simulink model "QiMotorController_ModelReference"  (R2021b)
settings: Solver=FixedStepDiscrete  StartTime=0.0  StopTime=5  RelTol=1e-3
PreLoadFcn:
  | RTWConfigurationCB('preloadfcn', bdroot);
PostLoadFcn:
  | load('configuration/data_struct.mat');
  | load('configuration/fluxMaps_propMotor.mat');
  | load('configuration/parameterInit_PROP.mat');
  | load('configuration/parameterInit_PUMP.mat');
  | load('configuration/parameterInit_PITCH.mat');
  | load('configuration/parameterInit_TILT.mat');
  | %load('configuration/base_workspace_signal_definition.mat');
  | %load('resolvedatastores_to_baseworkspace_for_faster_simulation.mat');
model workspace (MAT data in the model file):
  ADC_CALIBRATION_SAMPLES : Simulink.Parameter (value not decoded)
  DEFAULT_RESOLVER_CONTROL_WORD : Simulink.Parameter (value not decoded)
  PLL_FREQUENCY : Simulink.Parameter (value not decoded)
  SIMULATION_OPTIONS : Simulink.Parameter (value not decoded)
  TARGET_CODE_GEN : Simulink.Parameter (value not decoded)
  Ts = 2.5e-07
symbols that are objects in the model workspace (value not decoded): PLL_FREQUENCY, TARGET_CODE_GEN
undefined symbols (not defined in the file): DEADTIME_NS__PITCH, DEADTIME_NS__PROP, DEADTIME_NS__PUMP, DEADTIME_NS__TILT, fIa_, fIb_, fIc_, fIdc_, fMotorEncoderFloat_, fMotorSensorSpeed_, fUa_, fUb_, fUc_, fUdc_, inbtilt, mdl_pitch_uiAPUFlags, mdl_pitch_uiFlags, modelData, oMot_, oOut_, opInputResolverData_, oPitch, oState_, PLANT_SPEED_QUADRATIC_COEFF__PUMP, POLE_PAIRS_INIT__PITCH, POLE_PAIRS_INIT__PROP, POLE_PAIRS_INIT__PUMP, POLE_PAIRS_INIT__TILT, PWM_FREQ_KHZ__PITCH, PWM_FREQ_KHZ__PROP, PWM_FREQ_KHZ__PUMP, R_PHASE_INIT__PITCH, R_PHASE_INIT__PROP, R_PHASE_INIT__TILT, R_PHASE_INIT_PLANT__PUMP, uiControlReadback_, uiGateDriverStatus_
libraries: simulink x51, spsSeriesRLCBranchLib x25, spsMosfetLib x24, powerlib_extras x24, spsCurrentMeasurementLib x17, spsVoltageMeasurementLib x17, spsPermanentMagnetSynchronousMachineLib x3, spsDCVoltageSourceLib x2, motorModelLibrary x2, slpidlib x2, cstblocks x1, spspowerguiLib x1
(part 2 of 5)

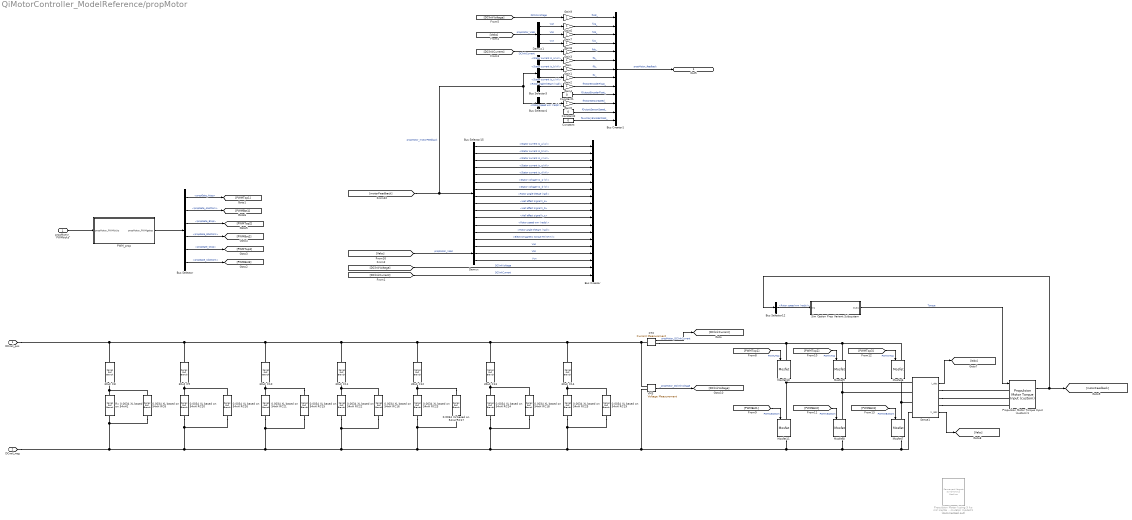
== system QiMotorController_ModelReference/propMotor ==
  propMotor_PWMticks : Inport
  0.0034 XL based on 54nH RC{8,15..19,26} (7 alike) : spsSeriesRLCBranchLib/Series RLC Branch  LConnTagsString=__new0  RConnTagsString=__new0  BranchType=R  Resistance=10000000  Inductance=33e-9  SetiL0=off  InitialCurrent=0  Capacitance=470e-6  Setx0=off  InitialVoltage=0  Measurements=None
  0.0034 XL based on 54nH RC{20..25} (6 alike) : spsSeriesRLCBranchLib/Series RLC Branch  LConnTagsString=__new0  RConnTagsString=__new0  BranchType=R  Resistance=0.0041  Inductance=33e-9  SetiL0=off  InitialCurrent=0  Capacitance=470e-6  Setx0=off  InitialVoltage=0  Measurements=None
  30uF C{8..10,12..14} (6 alike) : spsSeriesRLCBranchLib/Series RLC Branch  LConnTagsString=__new0  RConnTagsString=__new0  BranchType=C  Resistance=1  Inductance=1e-3  SetiL0=off  InitialCurrent=0  Capacitance=30e-6  Setx0=off  InitialVoltage=0  Measurements=Branch voltage and current
  30uF C11 : spsSeriesRLCBranchLib/Series RLC Branch  LConnTagsString=__new0  RConnTagsString=__new0  BranchType=C  Resistance=1  Inductance=1e-3  SetiL0=off  InitialCurrent=0  Capacitance=10e-6  Setx0=off  InitialVoltage=0  Measurements=Branch voltage and current
  Bus Creator : BusCreator  Inputs=19
  Bus Creator1 : BusCreator  Inputs=13  OutDataTypeStr=Bus: SAdcDataSingleIn_t
  Bus Selector : BusSelector  OutputSignals=propGate_Atop,propGate_Abottom,propGate_Btop,propGate_Bbottom,propGate_Ctop,propGate_Cbottom
  Bus Selector12 : BusSelector  OutputSignals=Rotor speed wm (rad/s)
  Bus Selector15 : BusSelector  OutputSignals=Stator current is_a (A),Stator current is_b (A),Stator current is_c (A),Stator current is_q (A),Stator current is_d (A),Stator voltage Vs_q (V),Stator voltage Vs_d (V),Rotor angle thetae (rad),Hall effect signal h_a,Hall effect signal h_b,Hall effect signal h_c,Rotor speed wm (rad/s),Rotor angle thetam (rad),Electromagnetic torque Te (N*m)
  Bus Selector3 : BusSelector  OutputSignals=Stator current is_a (A),Stator current is_b (A),Stator current is_c (A),Rotor angle thetam (rad)
  Bus Selector4 : BusSelector  OutputSignals=Rotor speed wm (rad/s)
  CT2 : spsCurrentMeasurementLib/Current Measurement  PhasorSimulation=off  OutputType=Complex  PSBequivalent=0
  Constant : Constant  Value=0  OutDataTypeStr=single
  Constant1 : Constant  Value=0  OutDataTypeStr=single
  Constant2 : Constant  Value=0  OutDataTypeStr=single
  Demux : Demux  Outputs=3
  Demux1 : Demux  Outputs=3
  Gain{,1..9} (10 alike) : Gain  OutDataTypeStr=single
  Mosfet{6..11} (6 alike) : spsMosfetLib/Mosfet  Ron=5e-3  Lon=0  Rd=0.01  Vfd=0  IC=0  Rs=1e5  Cs=inf  Measurements=on
  PWM_prop : Subsystem
  Propulsion Motor (using 5 kg m2 inertia consistent with the emulator model)1 : spsPermanentMagnetSynchronousMachineLib/Permanent Magnet Synchronous Machine  Commented=on  NbPhases=3  FluxDistribution=Sinusoidal  RotorType=Salient-pole  MechanicalLoad=Torque Tm  PresetModel=No  ShowDetailedParameters=on  MeasurementBus=off  Resistance=R_PHASE_INIT__PROP  Inductance=0  dqInductances=[160e-6 130e-6]  La=MOTOR_Ls  MachineConstant=Torque Constant (N.m / A_peak)  Flux=0.044127  VoltageCst=336.1575  TorqueCst=TORQUE_NM_PER_AMP_INIT__PROP  Flat=0  Mechanical=[0.89 0.005 POLE_PAIRS_INIT__PROP]  PolePairs=POLE_PAIRS_INIT__PROP  InitialConditions=[0,0,0,0]  InitialConditions5ph=[0 0 0 0 0 0]  RefAngle=Aligned with phase A axis (original Park)  IterativeDiscreteModel=Trapezoidal non iterative  TsBlock=Ts  TsPowergui=0
      link override From: GotoTag=tp8169b85b_15ba_4846_bb0f_92caecca5899
      settings: AttributesFormatString=\n
  Propulsion Motor Torque Input (custom)1 : motorModelLibrary/Propulsion Motor Torque Input (custom)  NbPhases=3  FluxDistribution=Sinusoidal  RotorType=Round  MechanicalLoad=Torque Tm  PresetModel=No  ShowDetailedParameters=on  MeasurementBus=off  Resistance=R_PHASE_INIT__PROP  Inductance=8.5e-3  dqInductances=[8.5e-3,8.5e-3]  La=LS_INIT__PROP  MachineConstant=Torque Constant (N.m / A_peak)  Flux=0.044127  VoltageCst=336.1575  TorqueCst=TORQUE_NM_PER_AMP_INIT__PROP  Flat=120  Mechanical=[0.89 0.005 POLE_PAIRS_INIT__PROP 0]  PolePairs=4  InitialConditions=[0,0, 0,0]  InitialConditions5ph=[0 0 0 0 0 0]  RefAngle=Aligned with phase A axis (original Park)  IterativeDiscreteModel=Trapezoidal non iterative  TsBlock=-1  TsPowergui=0
  Rx 0.0034 XL based on 54nH1 : spsSeriesRLCBranchLib/Series RLC Branch  LConnTagsString=__new0  RConnTagsString=__new0  BranchType=R  Resistance=0.0041  Inductance=33e-9  SetiL0=off  InitialCurrent=0  Capacitance=470e-6  Setx0=off  InitialVoltage=0  Measurements=None
  Sense1 : Subsystem
      settings: PortSchema="{\"entries\":[{\"content\":{\"sides\":[{\"content\":{\"connectorIds\":[\"LConn1\",\"LConn2\",\"LConn3\",\"LConn4\"]},\"type\":\"ConnectorPlacement.EquallySpacedRectSide\",\"uuid\":\"7842130e-3042-4aab-b72e-eb1cdec29ee8\"},{\"content\":{\"connectorIds\":[\"Out1\",\"RConn1\",\"RConn2\",\"RConn3\",\"Out2\"],\"side\":\"RIGHT\"},\"type\":\"ConnectorPlacement.EquallySpacedRectSide\",\"uuid\":\"c17ee381-f168-491a-818a-60a0284cb5f0\"},{\"content\":{\"connectorIds\":[],\"side\":\"TOP\"},\"type\":\"ConnectorPlacement.EquallySpacedRectSide\",\"uuid\":\"c745f3af-6fcc-4aa3-a9ef-8419a9649519\"}]},\"type\":\"ConnectorPlacement.EquallySpacedConnector\",\"uuid\":\"04fba2a7-cbbf-4a24-95eb-69eefae2f6e3\"}],\"packageUris\":[\"http://schema.mathworks.com/mf0/Connector/R2020b\"],\"version\":\"1.0\"}"
  Sim Option Prop Variant Subsystem : Subsystem  Variant=on
  VM3 : spsVoltageMeasurementLib/Voltage Measurement  PhasorSimulation=off  OutputType=Complex  PSBequivalent=0
  DCrail_pos : PMIOPort  Side=Left
  DCrail_neg : PMIOPort  Port=2  Side=Left
  Out5 : Outport  OutDataTypeStr=Bus: SAdcDataSingleIn_t
  wires:
  [PWMBot1] -> Mosfet11/1  "PWMUBottom"
  Sense1/1(I_abc) -> [Iabc]
  [PWMTop3] -> Mosfet6/1  "PWMWTop"
  [PWMBot2] -> Mosfet8/1  "PWMVBottom"
  [PWMTop2] -> Mosfet9/1  "PWMVTop"
  [PWMTop1] -> Mosfet10/1  "PWMUTop"
  [PWMBot3] -> Mosfet7/1  "PWMWBottom"
  Sense1/2(V_abc) -> [Vabc]
  Bus Selector/6 -> [PWMBot3]  "<propGate_Cbottom>"
  Bus Selector/5 -> [PWMTop3]  "<propGate_Ctop>"
  Bus Selector/1 -> [PWMTop1]  "<propGate_Atop>"
  Bus Selector/2 -> [PWMBot1]  "<propGate_Abottom>"
  Bus Selector/4 -> [PWMBot2]  "<propGate_Bbottom>"
  Bus Selector/3 -> [PWMTop2]  "<propGate_Btop>"
  Bus Selector15/7 -> Bus Creator/7  "<Stator voltage Vs_d (V)>"
  Bus Selector15/11 -> Bus Creator/11  "<Hall effect signal h_c>"
  Bus Selector15/5 -> Bus Creator/5  "<Stator current is_d (A)>"
  Bus Selector15/10 -> Bus Creator/10  "<Hall effect signal h_b>"
  Bus Selector15/9 -> Bus Creator/9  "<Hall effect signal h_a>"
  Bus Selector15/13 -> Bus Creator/13  "<Rotor angle thetam (rad)>"
  Bus Selector15/1 -> Bus Creator/1  "<Stator current is_a (A)>"
  Bus Selector15/8 -> Bus Creator/8  "<Rotor angle thetae (rad)>"
  Bus Selector15/2 -> Bus Creator/2  "<Stator current is_b (A)>"
  Bus Selector15/4 -> Bus Creator/4  "<Stator current is_q (A)>"
  Demux/2 -> Bus Creator/16  "Vbn"
  Demux/3 -> Bus Creator/17  "Vcn"
  Bus Selector15/12 -> Bus Creator/12  "<Rotor speed wm (rad/s)>"
  Bus Selector15/3 -> Bus Creator/3  "<Stator current is_c (A)>"
  [Vabc] -> Demux/1  "propMotor_Vabc"
  Bus Selector15/6 -> Bus Creator/6  "<Stator voltage Vs_q (V)>"
  Propulsion Motor Torque Input (custom)1/1 -> [motorFeedback], Bus Selector12/1
  propMotor_PWMticks/1 -> PWM_prop/1(propMotor_PWMticks)
  PWM_prop/1(propMotor_PWMgates) -> Bus Selector/1
  CT2/1 -> [DClinkCurrent]  "propMotor_DClinkCurrent"
  [DClinkCurrent] -> Bus Creator/19  "DClinkCurrent"
  VM3/1 -> [DClinkVoltage]  "_propMotor_DClinkVoltage"
  [DClinkVoltage] -> Bus Creator/18  "DClinkVoltage"
  Bus Selector12/1 -> Sim Option Prop Variant Subsystem/1(In1)  "<Rotor speed wm (rad/s)>"
  Sim Option Prop Variant Subsystem/1(Out1) -> Propulsion Motor Torque Input (custom)1/1  "Torque"
  Bus Selector15/14 -> Bus Creator/14  "<Electromagnetic torque Te (N*m)>"
  Demux/1 -> Bus Creator/15  "Van"
  Demux1/2 -> Gain7/1  "Vbn"
  Constant/1 -> Bus Creator1/13  "fAuxiliaryEncoderFloat_"
  Gain4/1 -> Bus Creator1/9  "fMotorEncoderFloat_"
  Gain9/1 -> Bus Creator1/1  "fUdc_"
  Gain6/1 -> Bus Creator1/2  "fUa_"
  Constant2/1 -> Bus Creator1/12  "fOutputSensorSpeed_"
  [Vabc] -> Demux1/1  "propMotor_Vabc"
  Gain2/1 -> Bus Creator1/8  "fIc_"
  Gain1/1 -> Bus Creator1/7  "fIb_"
  Gain7/1 -> Bus Creator1/3  "fUb_"
  Gain5/1 -> Bus Creator1/11  "fMotorSensorSpeed_"
  [motorFeedback] -> Bus Selector15/1, Bus Selector3/1, Bus Selector4/1  "propMotor_motorFeedback"
  Bus Creator1/1 -> Out5/1  "propMotor_feedback"
  Gain8/1 -> Bus Creator1/4  "fUc_"
  Gain3/1 -> Bus Creator1/5  "fIdc_"
  Demux1/3 -> Gain8/1  "Vcn"
  [DClinkVoltage] -> Gain9/1  "DClinkVoltage"
  Gain/1 -> Bus Creator1/6  "fIa_"
  Demux1/1 -> Gain6/1  "Van"
  Constant1/1 -> Bus Creator1/10  "fOutputEncoderFloat_"
  [DClinkCurrent] -> Gain3/1  "DClinkCurrent"
  Bus Selector3/3 -> Gain2/1  "<Stator current is_c (A)>"
  Bus Selector3/2 -> Gain1/1  "<Stator current is_b (A)>"
  Bus Selector3/1 -> Gain/1  "<Stator current is_a (A)>"
  Bus Selector3/4 -> Gain4/1  "<Rotor angle thetam (rad)>"
  Bus Selector4/1 -> Gain5/1  "<Rotor speed wm (rad/s)>"
  connections:
  Sense1/RConn1 -- Propulsion Motor Torque Input (custom)1/LConn1
  Sense1/RConn2 -- Propulsion Motor Torque Input (custom)1/LConn2
  Mosfet10/RConn1 -- Mosfet11/LConn1 -- Sense1/LConn1
  Sense1/RConn3 -- Propulsion Motor Torque Input (custom)1/LConn3
  Mosfet9/RConn1 -- Mosfet8/LConn1 -- Sense1/LConn2
  Mosfet6/RConn1 -- Mosfet7/LConn1 -- Sense1/LConn3
  0.0034 XL based on 54nH RC24/LConn1 -- 30uF C13/RConn1 -- 0.0034 XL based on 54nH RC18/LConn1
  0.0034 XL based on 54nH RC25/LConn1 -- 30uF C14/RConn1 -- 0.0034 XL based on 54nH RC19/LConn1
  0.0034 XL based on 54nH RC15/LConn1 -- 30uF C10/RConn1 -- 0.0034 XL based on 54nH RC21/LConn1
  Rx 0.0034 XL based on 54nH1/LConn1 -- 30uF C8/RConn1 -- 0.0034 XL based on 54nH RC8/LConn1
  0.0034 XL based on 54nH RC20/LConn1 -- 30uF C9/RConn1 -- 0.0034 XL based on 54nH RC26/LConn1
  0.0034 XL based on 54nH RC17/LConn1 -- 30uF C12/RConn1 -- 0.0034 XL based on 54nH RC23/LConn1
  0.0034 XL based on 54nH RC22/LConn1 -- 30uF C11/RConn1 -- 0.0034 XL based on 54nH RC16/LConn1
  Mosfet6/LConn1 -- CT2/RConn1 -- Mosfet10/LConn1 -- Mosfet9/LConn1
  Mosfet8/RConn1 -- Mosfet11/RConn1 -- VM3/LConn2 -- 0.0034 XL based on 54nH RC19/RConn1 -- 0.0034 XL based on 54nH RC25/RConn1 -- 0.0034 XL based on 54nH RC18/RConn1 -- 0.0034 XL based on 54nH RC24/RConn1 -- 0.0034 XL based on 54nH RC23/RConn1 -- 0.0034 XL based on 54nH RC17/RConn1 -- 0.0034 XL based on 54nH RC16/RConn1 -- 0.0034 XL based on 54nH RC22/RConn1 -- 0.0034 XL based on 54nH RC15/RConn1 -- 0.0034 XL based on 54nH RC21/RConn1 -- DCrail_neg/RConn1 -- 0.0034 XL based on 54nH RC8/RConn1 -- Rx 0.0034 XL based on 54nH1/RConn1 -- 0.0034 XL based on 54nH RC26/RConn1 -- 0.0034 XL based on 54nH RC20/RConn1 -- Mosfet7/RConn1 -- Sense1/LConn4
  30uF C13/LConn1 -- 30uF C9/LConn1 -- 30uF C8/LConn1 -- DCrail_pos/RConn1 -- 30uF C10/LConn1 -- 30uF C11/LConn1 -- 30uF C12/LConn1 -- CT2/LConn1 -- VM3/LConn1 -- 30uF C14/LConn1

== system QiMotorController_ModelReference/pumpfanMotor ==
  pumpMotor_PWMticks : Inport
  .45uF : spsSeriesRLCBranchLib/Series RLC Branch  LConnTagsString=__new0  RConnTagsString=__new0  BranchType=C  Resistance=1  Inductance=1e-3  SetiL0=off  InitialCurrent=0  Capacitance=0.45e-6  Setx0=off  InitialVoltage=0  Measurements=Branch voltage and current
  Affinity Law Tq Coeff: Inboard Fan : Constant  Commented=on  Value=PLANT_SPEED_QUADRATIC_COEFF__PUMP  SampleTime=-1
  Bus Creator : BusCreator  Inputs=19
  Bus Creator1 : BusCreator  Inputs=13  OutDataTypeStr=Bus: SAdcDataSingleIn_t
  Bus Selector : BusSelector  OutputSignals=pumpGate_Atop,pumpGate_Abottom,pumpGate_Btop,pumpGate_Bbottom,pumpGate_Ctop,pumpGate_Cbottom
  Bus Selector12 : BusSelector  OutputSignals=Rotor speed wm (rad/s)
  Bus Selector15 : BusSelector  OutputSignals=Stator current is_a (A),Stator current is_b (A),Stator current is_c (A),Stator current is_q (A),Stator current is_d (A),Stator voltage Vs_q (V),Stator voltage Vs_d (V),Rotor angle thetae (rad),Hall effect signal h_a,Hall effect signal h_b,Hall effect signal h_c,Rotor speed wm (rad/s),Rotor angle thetam (rad),Electromagnetic torque Te (N*m)
  Bus Selector3 : BusSelector  OutputSignals=Stator current is_a (A),Stator current is_b (A),Stator current is_c (A),Rotor angle thetam (rad)
  Bus Selector4 : BusSelector  OutputSignals=Rotor speed wm (rad/s)
  CT2 : spsCurrentMeasurementLib/Current Measurement  PhasorSimulation=off  OutputType=Complex  PSBequivalent=0
  Constant : Constant  Value=0  OutDataTypeStr=single
  Constant1 : Constant  Value=0  OutDataTypeStr=single
  Constant2 : Constant  Value=0  OutDataTypeStr=single
  Demux : Demux  Outputs=3
  Demux1 : Demux  Outputs=3
  Gain : Gain  Commented=on  Gain=1/(2*pi)*60
  Gain{1..10} (10 alike) : Gain  OutDataTypeStr=single
  Math Function1 : Math  Commented=on  Operator=square  SignedPower=on  SaturateOnIntegerOverflow=on
  Mosfet{6..11} (6 alike) : spsMosfetLib/Mosfet  Ron=5e-3  Lon=0  Rd=0.01  Vfd=0  IC=0  Rs=1e5  Cs=inf  Measurements=on
  PWM_pumpfan : Subsystem
  Product : Product  Commented=on
  Pumpfan Motor : motorModelLibrary/Permanent Magnet Synchronous Machine  NbPhases=3  FluxDistribution=Sinusoidal  RotorType=Round  MechanicalLoad=Torque Tm  PresetModel=No  ShowDetailedParameters=on  MeasurementBus=off  Resistance=R_PHASE_INIT_PLANT__PUMP  Inductance=8.5e-3  dqInductances=[8.5e-3,8.5e-3]  La=LS_INIT_PLANT_ARMATURE__PUMP  MachineConstant=Torque Constant (N.m / A_peak)  Flux=0.038  VoltageCst=68.9244  TorqueCst=TORQUE_NM_PER_AMP_INIT__PUMP  Flat=120  Mechanical=[0.9e-3 5e-5 POLE_PAIRS_INIT__PUMP 0]  PolePairs=4  InitialConditions=[0,0,0,0]  InitialConditions5ph=[0 0 0 0 0 0]  RefAngle=Aligned with phase A axis (original Park)  IterativeDiscreteModel=Trapezoidal non iterative  TsBlock=Ts  TsPowergui=0
  Sense1 : Subsystem
      settings: PortSchema="{\"entries\":[{\"content\":{\"sides\":[{\"content\":{\"connectorIds\":[\"LConn1\",\"LConn2\",\"LConn3\",\"LConn4\"]},\"type\":\"ConnectorPlacement.EquallySpacedRectSide\",\"uuid\":\"7842130e-3042-4aab-b72e-eb1cdec29ee8\"},{\"content\":{\"connectorIds\":[\"Out1\",\"RConn1\",\"RConn2\",\"RConn3\",\"Out2\"],\"side\":\"RIGHT\"},\"type\":\"ConnectorPlacement.EquallySpacedRectSide\",\"uuid\":\"c17ee381-f168-491a-818a-60a0284cb5f0\"},{\"content\":{\"connectorIds\":[],\"side\":\"TOP\"},\"type\":\"ConnectorPlacement.EquallySpacedRectSide\",\"uuid\":\"c745f3af-6fcc-4aa3-a9ef-8419a9649519\"}]},\"type\":\"ConnectorPlacement.EquallySpacedConnector\",\"uuid\":\"04fba2a7-cbbf-4a24-95eb-69eefae2f6e3\"}],\"packageUris\":[\"http://schema.mathworks.com/mf0/Connector/R2020b\"],\"version\":\"1.0\"}"
  Sim Option Pump Variant Subsystem : Subsystem  Variant=on
  VM3 : spsVoltageMeasurementLib/Voltage Measurement  PhasorSimulation=off  OutputType=Complex  PSBequivalent=0
  DCrail_pos : PMIOPort  Side=Left
  DCrail_neg : PMIOPort  Port=2  Side=Left
  Out5 : Outport  OutDataTypeStr=Bus: SAdcDataSingleIn_t
  wires:
  [PWMBot1] -> Mosfet11/1  "PWMUBottom"
  Sense1/1(I_abc) -> [Iabc]
  [PWMTop3] -> Mosfet6/1  "PWMWTop"
  [PWMBot2] -> Mosfet8/1  "PWMVBottom"
  [PWMTop2] -> Mosfet9/1  "PWMVTop"
  [PWMTop1] -> Mosfet10/1  "PWMUTop"
  [PWMBot3] -> Mosfet7/1  "PWMWBottom"
  Sense1/2(V_abc) -> [Vabc]
  Bus Selector/6 -> [PWMBot3]  "<pumpGate_Cbottom>"
  Bus Selector/5 -> [PWMTop3]  "<pumpGate_Ctop>"
  Bus Selector/1 -> [PWMTop1]  "<pumpGate_Atop>"
  Bus Selector/2 -> [PWMBot1]  "<pumpGate_Abottom>"
  Bus Selector/4 -> [PWMBot2]  "<pumpGate_Bbottom>"
  Bus Selector/3 -> [PWMTop2]  "<pumpGate_Btop>"
  Bus Selector15/7 -> Bus Creator/7  "<Stator voltage Vs_d (V)>"
  [motorFeedback] -> Bus Selector4/1, Bus Selector3/1, Bus Selector15/1
  Bus Selector15/5 -> Bus Creator/5  "<Stator current is_d (A)>"
  Bus Selector15/1 -> Bus Creator/1  "<Stator current is_a (A)>"
  Bus Selector15/2 -> Bus Creator/2  "<Stator current is_b (A)>"
  Bus Selector15/4 -> Bus Creator/4  "<Stator current is_q (A)>"
  Bus Selector15/3 -> Bus Creator/3  "<Stator current is_c (A)>"
  [Vabc] -> Demux/1
  Bus Selector15/6 -> Bus Creator/6  "<Stator voltage Vs_q (V)>"
  Bus Creator/1 -> ?  "pumpMotor_feedback"
  Pumpfan Motor/1 -> Bus Selector12/1, [motorFeedback]
  pumpMotor_PWMticks/1 -> PWM_pumpfan/1(pumpMotor_PWMticks)
  PWM_pumpfan/1(pumpMotor_PWMgates) -> Bus Selector/1
  CT2/1 -> [DClinkCurrent]  "DClinkCurrent"
  VM3/1 -> [DClinkVoltage]  "DClinkVoltage"
  Bus Selector12/1 -> Sim Option Pump Variant Subsystem/1(In1)  "<Rotor speed wm (rad/s)>"
  Sim Option Pump Variant Subsystem/1(Out1) -> Pumpfan Motor/1  "Torque"
  Math Function1/1 -> Product/1
  Gain/1 -> Math Function1/1
  Affinity Law Tq Coeff: Inboard Fan/1 -> Product/2
  Bus Selector15/8 -> Bus Creator/8  "<Rotor angle thetae (rad)>"
  Bus Selector15/9 -> Bus Creator/9  "<Hall effect signal h_a>"
  Bus Selector15/10 -> Bus Creator/10  "<Hall effect signal h_b>"
  Bus Selector15/11 -> Bus Creator/11  "<Hall effect signal h_c>"
  Bus Selector15/12 -> Bus Creator/12  "<Rotor speed wm (rad/s)>"
  Bus Selector15/13 -> Bus Creator/13  "<Rotor angle thetam (rad)>"
  Bus Selector15/14 -> Bus Creator/14  "<Electromagnetic torque Te (N*m)>"
  Demux/1 -> Bus Creator/15  "Van"
  Demux/2 -> Bus Creator/16  "Vbn"
  Demux/3 -> Bus Creator/17  "Vcn"
  [DClinkVoltage] -> Bus Creator/18  "DClinkVoltage"
  [DClinkCurrent] -> Bus Creator/19  "DClinkCurrent"
  Constant/1 -> Bus Creator1/13  "fAuxiliaryEncoderFloat_"
  Demux1/3 -> Gain9/1  "Vcn"
  Bus Selector4/1 -> Gain6/1  "<Rotor speed wm (rad/s)>"
  Bus Selector3/2 -> Gain2/1  "<Stator current is_b (A)>"
  Gain10/1 -> Bus Creator1/1  "fUdc_"
  Constant2/1 -> Bus Creator1/12  "fOutputSensorSpeed_"
  Bus Selector3/4 -> Gain5/1  "<Rotor angle thetam (rad)>"
  Bus Selector3/3 -> Gain3/1  "<Stator current is_c (A)>"
  Gain5/1 -> Bus Creator1/9  "fMotorEncoderFloat_"
  Gain9/1 -> Bus Creator1/4  "fUc_"
  Gain6/1 -> Bus Creator1/11  "fMotorSensorSpeed_"
  Gain3/1 -> Bus Creator1/8  "fIc_"
  Gain1/1 -> Bus Creator1/6  "fIa_"
  Gain8/1 -> Bus Creator1/3  "fUb_"
  Gain4/1 -> Bus Creator1/5  "fIdc_"
  Demux1/2 -> Gain8/1  "Vbn"
  Constant1/1 -> Bus Creator1/10  "fOutputEncoderFloat_"
  Bus Selector3/1 -> Gain1/1  "<Stator current is_a (A)>"
  Demux1/1 -> Gain7/1  "Van"
  Gain2/1 -> Bus Creator1/7  "fIb_"
  [Vabc] -> Demux1/1  "pumpMotor_Vabc"
  [DClinkVoltage] -> Gain10/1  "DClinkVoltage"
  [DClinkCurrent] -> Gain4/1  "DClinkCurrent"
  Gain7/1 -> Bus Creator1/2  "fUa_"
  Bus Creator1/1 -> Out5/1  "pumpMotor_feedback"
  connections:
  Pumpfan Motor/LConn1 -- Sense1/RConn1
  Pumpfan Motor/LConn2 -- Sense1/RConn2
  Mosfet10/RConn1 -- Mosfet11/LConn1 -- Sense1/LConn1
  Pumpfan Motor/LConn3 -- Sense1/RConn3
  Mosfet9/RConn1 -- Mosfet8/LConn1 -- Sense1/LConn2
  Mosfet6/RConn1 -- Mosfet7/LConn1 -- Sense1/LConn3
  Mosfet6/LConn1 -- Mosfet9/LConn1 -- CT2/RConn1 -- Mosfet10/LConn1
  Mosfet8/RConn1 -- Mosfet7/RConn1 -- Sense1/LConn4 -- Mosfet11/RConn1 -- .45uF/RConn1 -- DCrail_neg/RConn1 -- VM3/LConn2
  CT2/LConn1 -- DCrail_pos/RConn1 -- .45uF/LConn1 -- VM3/LConn1

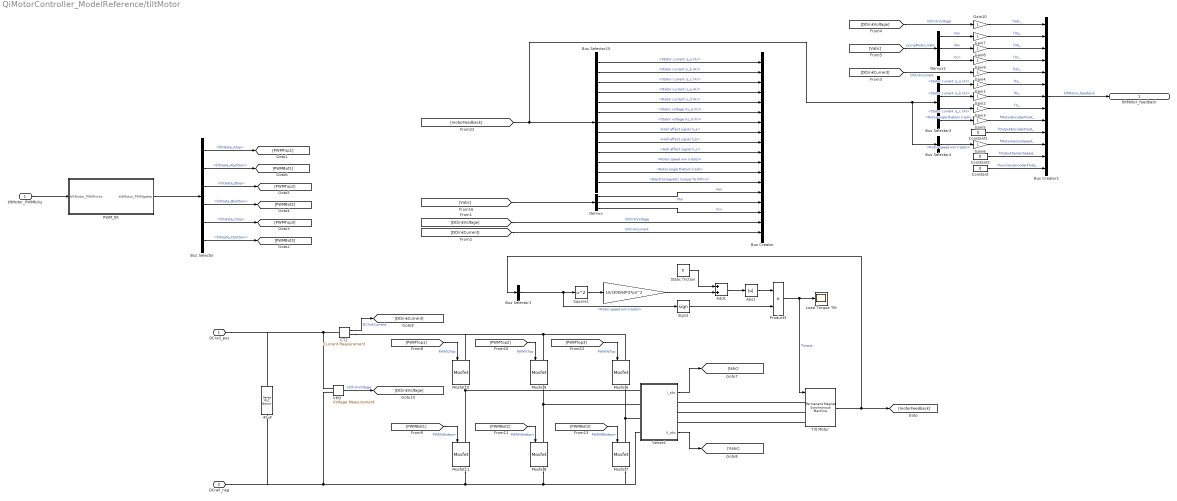
== system QiMotorController_ModelReference/tiltMotor ==
  tiltMotor_PWMticks : Inport
  " " : Gain  Gain=15/(300/60*2*pi)^2
  .45uF : spsSeriesRLCBranchLib/Series RLC Branch  LConnTagsString=__new0  RConnTagsString=__new0  BranchType=C  Resistance=1  Inductance=1e-3  SetiL0=off  InitialCurrent=0  Capacitance=.45e-6  Setx0=off  InitialVoltage=0  Measurements=Branch voltage and current
  Abs1 : Abs
  Add1 : Sum
  Bus Creator : BusCreator  Inputs=18
  Bus Creator1 : BusCreator  Inputs=13  OutDataTypeStr=Bus: SAdcDataSingleIn_t
  Bus Selector : BusSelector  OutputSignals=tiltGate_Atop,tiltGate_Abottom,tiltGate_Btop,tiltGate_Bbottom,tiltGate_Ctop,tiltGate_Cbottom
  Bus Selector1 : BusSelector  OutputSignals=Rotor speed wm (rad/s)
  Bus Selector15 : BusSelector  OutputSignals=Stator current is_a (A),Stator current is_b (A),Stator current is_c (A),Stator current is_q (A),Stator current is_d (A),Stator voltage Vs_q (V),Stator voltage Vs_d (V),Hall effect signal h_a,Hall effect signal h_b,Hall effect signal h_c,Rotor speed wm (rad/s),Rotor angle thetam (rad),Electromagnetic torque Te (N*m)
  Bus Selector3 : BusSelector  OutputSignals=Stator current is_a (A),Stator current is_b (A),Stator current is_c (A),Rotor angle thetam (rad)
  Bus Selector4 : BusSelector  OutputSignals=Rotor speed wm (rad/s)
  CT2 : spsCurrentMeasurementLib/Current Measurement  PhasorSimulation=off  OutputType=Complex  PSBequivalent=0
  Constant : Constant  Value=0  OutDataTypeStr=single
  Constant1 : Constant  Value=0  OutDataTypeStr=single
  Constant2 : Constant  Value=0  OutDataTypeStr=single
  Demux : Demux  Outputs=3
  Demux1 : Demux  Outputs=3
  Gain{1..10} (10 alike) : Gain  OutDataTypeStr=single
  Load Torque Tilt : Scope
  Mosfet{6..11} (6 alike) : spsMosfetLib/Mosfet  Ron=5e-3  Lon=0  Rd=0.01  Vfd=0  IC=0  Rs=1e5  Cs=inf  Measurements=on
  PWM_tilt : Subsystem
  Product3 : Product
  Sense1 : Subsystem
      settings: PortSchema="{\"entries\":[{\"content\":{\"sides\":[{\"content\":{\"connectorIds\":[\"LConn1\",\"LConn2\",\"LConn3\",\"LConn4\"]},\"type\":\"ConnectorPlacement.EquallySpacedRectSide\",\"uuid\":\"7842130e-3042-4aab-b72e-eb1cdec29ee8\"},{\"content\":{\"connectorIds\":[\"Out1\",\"RConn1\",\"RConn2\",\"RConn3\",\"Out2\"],\"side\":\"RIGHT\"},\"type\":\"ConnectorPlacement.EquallySpacedRectSide\",\"uuid\":\"c17ee381-f168-491a-818a-60a0284cb5f0\"},{\"content\":{\"connectorIds\":[],\"side\":\"TOP\"},\"type\":\"ConnectorPlacement.EquallySpacedRectSide\",\"uuid\":\"c745f3af-6fcc-4aa3-a9ef-8419a9649519\"}]},\"type\":\"ConnectorPlacement.EquallySpacedConnector\",\"uuid\":\"04fba2a7-cbbf-4a24-95eb-69eefae2f6e3\"}],\"packageUris\":[\"http://schema.mathworks.com/mf0/Connector/R2020b\"],\"version\":\"1.0\"}"
  Sign1 : Signum
  Square1 : Math  Operator=square  SaturateOnIntegerOverflow=on
  Static friction : Constant  Value=0  SampleTime=-1
  Tilt Motor : spsPermanentMagnetSynchronousMachineLib/Permanent Magnet Synchronous Machine  NbPhases=3  FluxDistribution=Sinusoidal  RotorType=Round  MechanicalLoad=Torque Tm  PresetModel=No  ShowDetailedParameters=on  MeasurementBus=off  Resistance=R_PHASE_INIT__TILT  Inductance=0  dqInductances=[160e-6 130e-6]  La=LS_INIT__TILT  MachineConstant=Torque Constant (N.m / A_peak)  Flux=0.15  VoltageCst=544.1398  TorqueCst=TORQUE_NM_PER_AMP_INIT__TILT  Flat=0  Mechanical=[0.01 0.005 POLE_PAIRS_INIT__TILT]  PolePairs=POLE_PAIRS_INIT__PROP  InitialConditions=[0,0,0,0]  InitialConditions5ph=[0 0 0 0 0 0]  RefAngle=Aligned with phase A axis (original Park)  IterativeDiscreteModel=Trapezoidal non iterative  TsBlock=Ts  TsPowergui=0
      link override From: GotoTag=tp8169b85b_15ba_4846_bb0f_92caecca5899
      settings: AttributesFormatString=\n
  VM3 : spsVoltageMeasurementLib/Voltage Measurement  PhasorSimulation=off  OutputType=Complex  PSBequivalent=0
  DCrail_pos : PMIOPort  Side=Left
  DCrail_neg : PMIOPort  Port=2  Side=Left
  tiltMotor_feedback : Outport  OutDataTypeStr=Bus: SAdcDataSingleIn_t
  wires:
  [PWMTop2] -> Mosfet9/1  "PWMVTop"
  [PWMBot3] -> Mosfet7/1  "PWMWBottom"
  Sense1/2(V_abc) -> [Vabc]
  [PWMBot1] -> Mosfet11/1  "PWMUBottom"
  [PWMTop1] -> Mosfet10/1  "PWMUTop"
  [PWMTop3] -> Mosfet6/1  "PWMWTop"
  Sense1/1(I_abc) -> [Iabc]
  [PWMBot2] -> Mosfet8/1  "PWMVBottom"
  Bus Selector/3 -> [PWMTop2]  "<tiltGate_Btop>"
  Bus Selector/1 -> [PWMTop1]  "<tiltGate_Atop>"
  Bus Selector/2 -> [PWMBot1]  "<tiltGate_Abottom>"
  Bus Selector/4 -> [PWMBot2]  "<tiltGate_Bbottom>"
  Bus Selector/6 -> [PWMBot3]  "<tiltGate_Cbottom>"
  Bus Selector/5 -> [PWMTop3]  "<tiltGate_Ctop>"
  Demux/3 -> Bus Creator/16  "Vcn"
  Bus Selector15/2 -> Bus Creator/2  "<Stator current is_b (A)>"
  Demux/1 -> Bus Creator/14  "Van"
  Demux/2 -> Bus Creator/15  "Vbn"
  Bus Selector15/12 -> Bus Creator/12  "<Rotor angle thetam (rad)>"
  Bus Selector15/13 -> Bus Creator/13  "<Electromagnetic torque Te (N*m)>"
  Bus Selector15/10 -> Bus Creator/10  "<Hall effect signal h_c>"
  Bus Selector15/8 -> Bus Creator/8  "<Hall effect signal h_a>"
  Bus Selector15/3 -> Bus Creator/3  "<Stator current is_c (A)>"
  Bus Selector15/11 -> Bus Creator/11  "<Rotor speed wm (rad/s)>"
  Bus Selector15/4 -> Bus Creator/4  "<Stator current is_q (A)>"
  Bus Selector15/6 -> Bus Creator/6  "<Stator voltage Vs_q (V)>"
  Bus Selector15/9 -> Bus Creator/9  "<Hall effect signal h_b>"
  Bus Selector15/5 -> Bus Creator/5  "<Stator current is_d (A)>"
  Bus Selector15/1 -> Bus Creator/1  "<Stator current is_a (A)>"
  Bus Selector15/7 -> Bus Creator/7  "<Stator voltage Vs_d (V)>"
  [Vabc] -> Demux/1
  PWM_tilt/1(tiltMotor_PWMgates) -> Bus Selector/1
  tiltMotor_PWMticks/1 -> PWM_tilt/1(tiltMotor_PWMticks)
  CT2/1 -> [DClinkCurrent]  "DClinkCurrent"
  VM3/1 -> [DClinkVoltage]  "DClinkVoltage"
  [DClinkCurrent] -> Bus Creator/18  "DClinkCurrent"
  [DClinkVoltage] -> Bus Creator/17  "DClinkVoltage"
  Add1/1 -> Abs1/1
  Abs1/1 -> Product3/1
  Tilt Motor/1 -> Bus Selector1/1, [motorFeedback]
  Bus Selector1/1 -> Sign1/1, Square1/1  "<Rotor speed wm (rad/s)>"
  Product3/1 -> Tilt Motor/1, Load Torque Tilt/1  "Torque"
  Static friction/1 -> Add1/1
  Square1/1 -> " "/1
  " "/1 -> Add1/2
  Sign1/1 -> Product3/2
  Bus Selector3/3 -> Gain3/1  "<Stator current is_c (A)>"
  Bus Selector3/1 -> Gain1/1  "<Stator current is_a (A)>"
  [DClinkVoltage] -> Gain10/1  "DClinkVoltage"
  [DClinkCurrent] -> Gain4/1  "DClinkCurrent"
  Demux1/2 -> Gain8/1  "Vbn"
  Gain6/1 -> Bus Creator1/11  "fMotorSensorSpeed_"
  [motorFeedback] -> Bus Selector4/1, Bus Selector3/1, Bus Selector15/1
  Gain2/1 -> Bus Creator1/7  "fIb_"
  Demux1/1 -> Gain7/1  "Van"
  Gain9/1 -> Bus Creator1/4  "fUc_"
  Bus Selector4/1 -> Gain6/1  "<Rotor speed wm (rad/s)>"
  [Vabc] -> Demux1/1  "pumpMotor_Vabc"
  Bus Selector3/2 -> Gain2/1  "<Stator current is_b (A)>"
  Constant2/1 -> Bus Creator1/12  "fOutputSensorSpeed_"
  Bus Selector3/4 -> Gain5/1  "<Rotor angle thetam (rad)>"
  Gain1/1 -> Bus Creator1/6  "fIa_"
  Constant/1 -> Bus Creator1/13  "fAuxiliaryEncoderFloat_"
  Gain7/1 -> Bus Creator1/2  "fUa_"
  Gain4/1 -> Bus Creator1/5  "fIdc_"
  Gain3/1 -> Bus Creator1/8  "fIc_"
  Gain5/1 -> Bus Creator1/9  "fMotorEncoderFloat_"
  Constant1/1 -> Bus Creator1/10  "fOutputEncoderFloat_"
  Demux1/3 -> Gain9/1  "Vcn"
  Gain10/1 -> Bus Creator1/1  "fUdc_"
  Gain8/1 -> Bus Creator1/3  "fUb_"
  Bus Creator1/1 -> tiltMotor_feedback/1  "tiltMotor_feedback"
  connections:
  Mosfet6/LConn1 -- Mosfet10/LConn1 -- CT2/RConn1 -- Mosfet9/LConn1
  Mosfet11/RConn1 -- .45uF/RConn1 -- DCrail_neg/RConn1 -- VM3/LConn2 -- Mosfet8/RConn1 -- Mosfet7/RConn1 -- Sense1/LConn4
  Mosfet7/LConn1 -- Sense1/LConn3 -- Mosfet6/RConn1
  Mosfet8/LConn1 -- Sense1/LConn2 -- Mosfet9/RConn1
  Mosfet11/LConn1 -- Sense1/LConn1 -- Mosfet10/RConn1
  Tilt Motor/LConn1 -- Sense1/RConn1
  Tilt Motor/LConn2 -- Sense1/RConn2
  Tilt Motor/LConn3 -- Sense1/RConn3
  CT2/LConn1 -- .45uF/LConn1 -- DCrail_pos/RConn1 -- VM3/LConn1

== system QiMotorController_ModelReference/Encoder1/1//T Simulation ==
  In3 : Inport
  1 : Constant  Value=30  OutDataTypeStr=uint32  SampleTime=-1
  2 : Constant  Value=30  OutDataTypeStr=uint32  SampleTime=-1
  3 : Constant  Value=0  OutDataTypeStr=uint32  SampleTime=-1
  Add : Sum  OutDataTypeStr=uint32
  Data Type Conversion : DataTypeConversion  OutDataTypeStr=uint32
  Data Type Conversion1 : DataTypeConversion  OutDataTypeStr=uint32
  Detect Rise Positive : simulink/Logic and Bit Operations/Detect Rise Positive  vinit=0  OutDataTypeStr=boolean
  Product : Product  OutDataTypeStr=uint32  RndMeth=Zero
  Product1 : Product  OutDataTypeStr=uint32  RndMeth=Zero
  Rate Transition : RateTransition  OutPortSampleTimeOpt=Multiple of input port sample time  OutPortSampleTimeMultiple=2
  Rate Transition1 : RateTransition  OutPortSampleTimeMultiple=2
  Rate Transition2 : RateTransition
  Rate Transition3 : RateTransition  OutPortSampleTimeMultiple=-1
  Rate Transition4 : RateTransition  OutPortSampleTimeOpt=Multiple of input port sample time  OutPortSampleTimeMultiple=2
  Rate Transition5 : RateTransition  OutPortSampleTimeMultiple=2
  Rate Transition6 : RateTransition  OutPortSampleTimeMultiple=-1
  Scope1 : Scope  Commented=on  NumInputPorts=4
  Scope2 : Scope  Commented=on  NumInputPorts=4
  Source Clock : DiscretePulseGenerator  PulseType=Time based  Period=30/PLL_FREQUENCY  PulseWidth=50
  Switch1 : Switch  Criteria=u2 > Threshold
  Switch2 : Switch  Criteria=u2 > Threshold
  Out1 : Outport
  Out2 : Outport  Port=2
  wires:
  Source Clock/1 -> [Clock], Add/1, Scope1/4
  [ResetCounter] -> Scope1/2, Switch1/2
  3/1 -> Switch1/1
  Switch1/1 -> Add/2, Scope1/3
  Detect Rise Positive/1 -> [ResetCounter]
  Rate Transition/1 -> Rate Transition1/1
  Add/1 -> Rate Transition/1
  [ResetCounter] -> Scope2/3, Switch2/2
  Data Type Conversion/1 -> Out1/1  "PM_qcprd"
  Rate Transition1/1 -> Scope1/1, Switch1/3, Product1/1, Switch2/1, Scope2/2
  [Clock] -> Scope2/4
  In3/1 -> Rate Transition2/1
  Rate Transition2/1 -> Detect Rise Positive/1
  Switch2/1 -> Product/1, Rate Transition4/1, Scope2/1
  1/1 -> Product/2
  Rate Transition4/1 -> Rate Transition5/1
  Rate Transition5/1 -> Switch2/3
  2/1 -> Product1/2
  Data Type Conversion1/1 -> Out2/1  "PM_qctmr"
  Product/1 -> Rate Transition3/1
  Product1/1 -> Rate Transition6/1
  Rate Transition3/1 -> Data Type Conversion/1
  Rate Transition6/1 -> Data Type Conversion1/1

== system QiMotorController_ModelReference/FPGA Feedback for Sim/pitchMotor ==
  Bus Creator : BusCreator  Inputs=4
  Constant : Constant  Value=0x61  OutDataTypeStr=uint32  SampleTime=-1
  Constant1 : Constant  Value=0  OutDataTypeStr=uint32  SampleTime=-1
  Constant2 : Constant  Value=0  OutDataTypeStr=uint32  SampleTime=-1
  Constant3 : Constant  Value=0  OutDataTypeStr=uint32  SampleTime=-1
  Out1 : Outport
  wires:
  Constant2/1 -> Bus Creator/1  "oPitch.oMot_.oOut_.uiGateDriverStatus_"
  Bus Creator/1 -> Out1/1  "pitchMotor_FPGAfeedback"
  Constant1/1 -> Bus Creator/2  "mdl_pitch_uiFlags"
  Constant3/1 -> Bus Creator/3  "mdl_pitch_uiAPUFlags"
  Constant/1 -> Bus Creator/4  "oPitch.oMot_.oState_.opInputResolverData_.uiControlReadback_"

== system QiMotorController_ModelReference/FPGA Feedback for Sim/tiltMotor ==
  Bus Creator : BusCreator  Inputs=6
  Constant : Constant  Value=0x61  OutDataTypeStr=uint32  SampleTime=-1
  Constant1 : Constant  Value=0  OutDataTypeStr=uint32  SampleTime=-1
  Constant2 : Constant  Value=0  OutDataTypeStr=uint32  SampleTime=-1
  Constant3 : Constant  Value=0  OutDataTypeStr=uint32  SampleTime=-1
  Constant6 : Constant  Value=0x4  OutDataTypeStr=uint32  SampleTime=-1
  Constant7 : Constant  OutDataTypeStr=uint32  SampleTime=-1
  Out1 : Outport
  wires:
  Constant2/1 -> Bus Creator/1  "oTilt.oMot_.oOut_.uiGateDriverStatus_"
  Bus Creator/1 -> Out1/1  "tiltMotor_FPGAfeedback"
  Constant1/1 -> Bus Creator/2  "mdl_tilt_uiFlags"
  Constant3/1 -> Bus Creator/3  "mdl_tilt_uiAPUFlags"
  Constant/1 -> Bus Creator/4  "oTilt.oMot_.oState_.opInputResolverData_.uiControlReadback_"
  Constant6/1 -> Bus Creator/5  "mdl_tilt_uiInputSensorFlags"
  Constant7/1 -> Bus Creator/6  "mdl_tilt_uiOutputSensorFlags"

== system QiMotorController_ModelReference/Fault Injection/pitchMotor_faults ==
  note: 10Hz
      | Change the "Sim Disturbance" value from zero to the desired DC bus simulated voltage (only changes what the sensor would see, not the actual bus voltage).
      | Should see:
      | 1. DC bus voltage increases or decreases when the command is applied.
      | 2. Within 0.1s, PWM commands should go to zero.
      | 3. After another 0.1s, the uiDriveState should move to 1003 (low) or 1004 (high).
      | Currently there is no fault clear for simulation (11/17/21), though that functionality should be added.
  note: 200Hz
      | Change the "Sim Disturbance" value from zero to the desired DC bus simulated current (only changes what the sensor would see, not the actual current).
      | Should see:
      | 1. DC bus current increases or decreases when the command is applied.
      | 2. Within 0.005s, PWM commands should go to zero.
      | 3. After another 0.0.005s, the uiDriveState should move to 1006 (low) or 1005 (high).
      | Currently there is no fault clear for simulation (11/18/21), though that functionality should be added.
  note: 20kHz
      | Change the "Sim Disturbance" value from zero to the desired simulated phase current magnitude (only changes what is calculated from the sensor, not the actual current). When the change from zero is detected, the value is written to the target phase (with -0.5 * that value written to the other 2 phases to maintain Kirchoff's law and prevent a 1034 fault trip). Target_phase: 1=A, 2=B, 3=C.
      | Should see:
      | 1. Calculated current magnitude increases when the command is applied.
      | 2. Within 0.1s, PWM commands should go to zero.
      | 3. After another 0.1s, the uiDriveState should move to 1007.
      | Currently there is no fault clear for simulation (11/17/21), though that functionality should be added.
      |
      | VP target for 1007: 8.5A +- 0.5A
      | VP target for 1008: 10A +- 0.1A
      |
      | Because the auxiliary voltage trip codes can only be accessed (in the MBD code) once a 1007 fault has been detected, the test cases for 1034-1039 faults are included within the "Phase Current Disturbance" block.
      |
      | Similarly, the 1015 fault (software watchdog timer) can only be triggered in the MBD code once a 1007 has been detected, that test case is included here as well.
  pitchMotor_feedback : Inport  OutDataTypeStr=Bus: SAdcDataSingleIn_t
  pitchMotor_FPGAfeedback : Inport  Port=2
  Bus Assignment : BusAssignment  AssignedSignals=fUdc_,fIdc_,fIa_,fIb_,fIc_
  Bus Assignment1 : BusAssignment  AssignedSignals=oPitch:oMot_:oOut_:uiGateDriverStatus_,mdl_pitch_uiFlags,mdl_pitch_uiAPUFlags,oPitch:oMot_:oState_:opInputResolverData_:uiControlReadback_
  Bus Selector : BusSelector  OutputSignals=fUdc_
  Bus Selector1 : BusSelector  OutputSignals=fIdc_
  Bus Selector2 : BusSelector  OutputSignals=fIa_,fIb_,fIc_
  Bus Selector3 : BusSelector  OutputSignals=oPitch:oMot_:oOut_:uiGateDriverStatus_
  Bus Selector4 : BusSelector  OutputSignals=mdl_pitch_uiFlags
  Bus Selector5 : BusSelector  OutputSignals=mdl_pitch_uiAPUFlags
  Bus Selector6 : BusSelector  OutputSignals=oPitch:oMot_:oState_:opInputResolverData_:uiControlReadback_
  DC Current Disturbance : Subsystem  TreatAsAtomicUnit=on
  DC Voltage Disturbance : Subsystem  TreatAsAtomicUnit=on
  Demux : Demux  Outputs=3
  Mux : Mux  Inputs=3
  Phase Current & Aux Disturbances : Subsystem  TreatAsAtomicUnit=on
  Position Control Disturbances : Subsystem  TreatAsAtomicUnit=on
  Rate Transition : RateTransition
  Rate Transition11 : RateTransition
  Sim Disturbance Pitch Motor IPhaseMagnitude : Constant  Value=0  OutDataTypeStr=single  SampleTime=-1
  Sim Disturbance Pitch Motor Idc : Constant  Value=0  OutDataTypeStr=single  SampleTime=-1
  Sim Disturbance Pitch Motor Udc : Constant  Value=0  OutDataTypeStr=single  SampleTime=-1
  Sim Disturbance Pitch Motor inputResolver_uiControlFeedback : Constant  Value=0  OutDataTypeStr=uint32  SampleTime=-1
  auxTripCode(0,1015,1017,1018,1034-1039) : Constant  Value=0  OutDataTypeStr=uint32  SampleTime=-1
  phaseCode(1=A,2=B,3=C) : Constant  OutDataTypeStr=uint32  SampleTime=-1
  motorMeasure_pitch : Outport  OutDataTypeStr=Bus: SAdcDataSingleIn_t
  fpgaFeedback_pitch : Outport  Port=2
  wires:
  Sim Disturbance Pitch Motor Udc/1 -> DC Voltage Disturbance/2(Udc_value)
  Bus Selector/1 -> DC Voltage Disturbance/1(Udc_feedback)  "<fUdc_>"
  DC Voltage Disturbance/1(Udc_fault) -> Bus Assignment/2
  Bus Assignment/1 -> motorMeasure_pitch/1
  Sim Disturbance Pitch Motor Idc/1 -> DC Current Disturbance/2(Idc_value)
  Bus Selector1/1 -> DC Current Disturbance/1(Idc_feedback)  "<fIdc_>"
  DC Current Disturbance/1(Idc_fault) -> Bus Assignment/3
  Sim Disturbance Pitch Motor IPhaseMagnitude/1 -> Phase Current & Aux Disturbances/2(IphMagnitude_value)
  Mux/1 -> Phase Current & Aux Disturbances/1(Iabc_feedback)
  Bus Selector2/1 -> Mux/1  "<fIa_>"
  Bus Selector2/2 -> Mux/2  "<fIb_>"
  Bus Selector2/3 -> Mux/3  "<fIc_>"
  phaseCode(1=A,2=B,3=C)/1 -> Phase Current & Aux Disturbances/3(Target_phase)
  Demux/1 -> Bus Assignment/4
  Demux/2 -> Bus Assignment/5
  Demux/3 -> Bus Assignment/6
  Phase Current & Aux Disturbances/1(Iabc_fault) -> Demux/1
  Bus Selector3/1 -> Phase Current & Aux Disturbances/5(uiGateDriverStatus)  "<oPitch:oMot_:oOut_:uiGateDriverStatus_>"
  pitchMotor_FPGAfeedback/1 -> Bus Selector3/1, Bus Selector4/1, Bus Selector5/1, Bus Selector6/1, Rate Transition/1
  Bus Assignment1/1 -> fpgaFeedback_pitch/1
  auxTripCode(0,1015,1017,1018,1034-1039)/1 -> Phase Current & Aux Disturbances/4(Aux_trip_code)
  Bus Selector4/1 -> Phase Current & Aux Disturbances/6(mdl_pitch_uiFlags)  "<mdl_pitch_uiFlags>"
  Phase Current & Aux Disturbances/3(uiFlags_fault) -> Bus Assignment1/3
  Phase Current & Aux Disturbances/4(uiAPUFlags_fault) -> Bus Assignment1/4
  Bus Selector5/1 -> Phase Current & Aux Disturbances/7(mdl_pitch_uiAPUFlags)  "<mdl_pitch_uiAPUFlags>"
  Phase Current & Aux Disturbances/2(uiGateDriverStatus_fault) -> Bus Assignment1/2
  Bus Selector6/1 -> Position Control Disturbances/1(uiControlFeedback)  "<oPitch:oMot_:oState_:opInputResolverData_:uiControlReadback_>"
  Sim Disturbance Pitch Motor inputResolver_uiControlFeedback/1 -> Position Control Disturbances/2(uiControlFeedback_value)
  Position Control Disturbances/1(uiControlFeedback_fault) -> Bus Assignment1/5
  pitchMotor_feedback/1 -> Rate Transition11/1, Bus Selector/1, Bus Selector1/1, Bus Selector2/1
  Rate Transition11/1 -> Bus Assignment/1
  Rate Transition/1 -> Bus Assignment1/1

== system QiMotorController_ModelReference/InboardTiltDragLaw2/Subsystem1 ==
  Bus Element In3 : Inport  PortName=torque_load
  In Bus Element : Inport  Port=2  PortName=DrgMlt
  In Bus Element1 : Inport  Port=3  PortName=n_inv
  MATLAB Function : MATLAB Function  TreatAsAtomicUnit=on
  Product : Product  Inputs=3
  Reciprocal : Product  Inputs=/
  Reciprocal1 : Product  Inputs=/
  VelocityRatio : Constant  Value=161  OutDataTypeStr=single  SampleTime=1e-2
  Bus Element Out : Outport  PortName=torque_load_m
  wires:
  Reciprocal1/1 -> Product/3
  MATLAB Function/1(Eta) -> Reciprocal1/1
  In Bus Element1/1 -> MATLAB Function/2(n_inv)
  In Bus Element/1 -> MATLAB Function/1(DrgMlt)
  VelocityRatio/1 -> Reciprocal/1
  Bus Element In3/1 -> Product/2
  Product/1 -> Bus Element Out/1
  Reciprocal/1 -> Product/1

== system QiMotorController_ModelReference/InboardTiltDragLaw2/drag2 ==
  Bus Element In10 : Inport  PortName=torque_out_m
  Bus Element In3 : Inport  Port=2  PortName=velocity_m
  Bus Element In11 : Inport  Port=2  PortName=velocity_m
  Bus Element In4 : Inport  Port=2  PortName=velocity_m
  Bus Element In12 : Inport  Port=3  PortName=motor_temp
  Bus Element In15 : Inport  Port=4  PortName=torque_load_m
  Bus Element In9 : Inport  Port=4  PortName=torque_load_m
  Bus Element In6 : Inport  Port=5  PortName=n_invs
  In Bus Element : Inport  Port=6  PortName=DrgMlt
  In Bus Element1 : Inport  Port=6  PortName=DrgMlt
  In Bus Element2 : Inport  Port=6  PortName=DrgMlt
  Abs3 : Abs
  Abs6 : Abs
  Add : Sum
  Add1 : Sum
  Display : Display
  Gain1 : Gain  Gain=-1
  PhaseShortDrag : Constant  Value=0  OutDataTypeStr=Inherit: Inherit via back propagation
  Product1 : Product
  Saturation : Saturate  UpperLimit=100  LowerLimit=0
  Saturation2 : Saturate  UpperLimit=70  LowerLimit=0
  Switch : Switch
  Switch1 : Switch  Criteria=u2 > Threshold
  Unary Minus1 : UnaryMinus
  Zero : Constant  Value=0  OutDataTypeStr=Inherit: Inherit via back propagation
  coulomb_drag_logic : Subsystem
  friction : Lookup_n-D  BreakpointsForDimension1=inbtilt.DragTemperatureBreakpoints  BreakpointsForDimension2=inbtilt.DragSpeedBreakpoints  Table=inbtilt.DragTorqueTable  InternalRulePriority=Speed  RndMeth=Simplest  InputSameDT=on
      settings: InputPortMap=u0,u1
  load : Subsystem
  Out Bus Element : Outport  PortName=drag_torque
  Bus Element Out : Outport  Port=2  PortName=load_torque
  wires:
  In Bus Element1/1 -> Switch1/2
  In Bus Element2/1 -> Saturation/1
  In Bus Element/1 -> Switch/2
  Bus Element In12/1 -> Saturation2/1
  Saturation/1 -> Product1/2
  Zero/1 -> Switch/3
  Switch1/1 -> Unary Minus1/1
  Bus Element In9/1 -> Switch1/3
  friction/1 -> Product1/1  "nominal_drag"
  PhaseShortDrag/1 -> Add/2
  Abs6/1 -> coulomb_drag_logic/2(net_torque_m)  "nettq"
  Bus Element In15/1 -> load/2(ideal_load_torque_m)
  Bus Element In6/1 -> load/4(n_invs)
  Unary Minus1/1 -> Add1/2, Bus Element Out/1
  Bus Element In11/1 -> load/1(velocity_m)
  coulomb_drag_logic/1(drag_torque_out_m) -> Gain1/1  "drag"
  Add/1 -> Out Bus Element/1
  Abs3/1 -> friction/2
  Bus Element In3/1 -> Abs3/1
  Bus Element In10/1 -> Add1/1
  Add1/1 -> Abs6/1
  Gain1/1 -> Switch/1
  Saturation2/1 -> load/3(motor_temp), friction/1  "T"
  load/1(load_torque) -> Switch1/1, Display/1
  Switch/1 -> Add/1
  Bus Element In4/1 -> coulomb_drag_logic/1(velocity_m)
  Product1/1 -> coulomb_drag_logic/3(nominal_drag_torque_m)  "nominal_drag"

== system QiMotorController_ModelReference/Signal Conditioning/qi_dsm_to_sinc1 ==
  test_signal : Inport
  compute_dsm_output : Subsystem
  compute_sinc3_output : Subsystem
  out_sig : Outport
  wires:
  test_signal/1 -> compute_dsm_output/1(sig_in)
  compute_sinc3_output/1(out_sig) -> out_sig/1
  compute_dsm_output/1(pdm_signal) -> compute_sinc3_output/1(bp_signal)

== system QiMotorController_ModelReference/Signal Conditioning/qi_dsm_to_sinc2 ==
  test_signal : Inport
  compute_dsm_output : Subsystem
  compute_sinc3_output : Subsystem
  out_sig : Outport
  wires:
  test_signal/1 -> compute_dsm_output/1(sig_in)
  compute_sinc3_output/1(out_sig) -> out_sig/1
  compute_dsm_output/1(pdm_signal) -> compute_sinc3_output/1(bp_signal)

== system QiMotorController_ModelReference/Signal Conditioning/qi_dsm_to_sinc3 ==
  test_signal : Inport
  compute_dsm_output : Subsystem
  compute_sinc3_output : Subsystem
  out_sig : Outport
  wires:
  test_signal/1 -> compute_dsm_output/1(sig_in)
  compute_sinc3_output/1(out_sig) -> out_sig/1
  compute_dsm_output/1(pdm_signal) -> compute_sinc3_output/1(bp_signal)

== system QiMotorController_ModelReference/Signal Conditioning/qi_dsm_to_sinc4 ==
  test_signal : Inport
  compute_dsm_output : Subsystem
  compute_sinc3_output : Subsystem
  out_sig : Outport
  wires:
  test_signal/1 -> compute_dsm_output/1(sig_in)
  compute_sinc3_output/1(out_sig) -> out_sig/1
  compute_dsm_output/1(pdm_signal) -> compute_sinc3_output/1(bp_signal)

== system QiMotorController_ModelReference/Signal Conditioning/qi_dsm_to_sinc5 ==
  test_signal : Inport
  compute_dsm_output : Subsystem
  compute_sinc3_output : Subsystem
  out_sig : Outport
  wires:
  test_signal/1 -> compute_dsm_output/1(sig_in)
  compute_sinc3_output/1(out_sig) -> out_sig/1
  compute_dsm_output/1(pdm_signal) -> compute_sinc3_output/1(bp_signal)

== system QiMotorController_ModelReference/Signal Conditioning/qi_dsm_to_sinc6 ==
  test_signal : Inport
  compute_dsm_output : Subsystem
  compute_sinc3_output : Subsystem
  out_sig : Outport
  wires:
  test_signal/1 -> compute_dsm_output/1(sig_in)
  compute_sinc3_output/1(out_sig) -> out_sig/1
  compute_dsm_output/1(pdm_signal) -> compute_sinc3_output/1(bp_signal)

== system QiMotorController_ModelReference/Signal Conditioning/qi_dsm_to_sinc7 ==
  test_signal : Inport
  compute_dsm_output : Subsystem
  compute_sinc3_output : Subsystem
  out_sig : Outport
  wires:
  test_signal/1 -> compute_dsm_output/1(sig_in)
  compute_sinc3_output/1(out_sig) -> out_sig/1
  compute_dsm_output/1(pdm_signal) -> compute_sinc3_output/1(bp_signal)

== system QiMotorController_ModelReference/Signal Conditioning/qi_dsm_to_sinc8 ==
  test_signal : Inport
  compute_dsm_output : Subsystem
  compute_sinc3_output : Subsystem
  out_sig : Outport
  wires:
  test_signal/1 -> compute_dsm_output/1(sig_in)
  compute_sinc3_output/1(out_sig) -> out_sig/1
  compute_dsm_output/1(pdm_signal) -> compute_sinc3_output/1(bp_signal)

== system QiMotorController_ModelReference/Simulation Controls/pitchMotor ==
  note: 1: Current controller
      | 2: Speed controller
      | 3: Position controller
  Bus Creator : BusCreator  Inputs=6
  pitchMotor_OneOverSensorPolepairs : Constant  OutDataTypeStr=single  SampleTime=-1
  pitchMotor_controlSelector : Constant  Value=3  OutDataTypeStr=uint32  SampleTime=-1
  pitchMotor_currentSetpoint : Constant  Value=1.5  OutDataTypeStr=single  SampleTime=-1
  pitchMotor_positionSetpoint : Step  Time=1.5  Before=pi/4  After=-pi/2  OutDataTypeStr=single
  pitchMotor_speedSetpoint : Constant  Value=1000  OutDataTypeStr=single  SampleTime=-1
  pitchMotor_uiEnable : Constant  OutDataTypeStr=uint32  SampleTime=-1
  Out1 : Outport
  wires:
  Bus Creator/1 -> Out1/1  "pitchMotor_simControls"
  pitchMotor_uiEnable/1 -> Bus Creator/1  "uiEnable"
  pitchMotor_controlSelector/1 -> Bus Creator/2  "controlSelector"
  pitchMotor_currentSetpoint/1 -> Bus Creator/3  "currentSetpoint"
  pitchMotor_speedSetpoint/1 -> Bus Creator/4  "speedSetpoint"
  pitchMotor_positionSetpoint/1 -> Bus Creator/5  "positionSetpoint"
  pitchMotor_OneOverSensorPolepairs/1 -> Bus Creator/6  "OneOverSensorPolePairs"

== system QiMotorController_ModelReference/Simulation Controls/propMotor ==
  Bus Creator : BusCreator  Inputs=1
  propMotor_uiEnable : Constant  OutDataTypeStr=uint32  SampleTime=-1
  Out1 : Outport
  wires:
  Bus Creator/1 -> Out1/1  "propMotor_simControls"
  propMotor_uiEnable/1 -> Bus Creator/1  "uiEnable"

== system QiMotorController_ModelReference/Simulation Controls/pumpMotor ==
  Bus Creator : BusCreator  Inputs=1
  pumpMotor_uiEnable : Constant  OutDataTypeStr=uint32  SampleTime=-1
  Out1 : Outport
  wires:
  Bus Creator/1 -> Out1/1  "pumpMotor_simControls"
  pumpMotor_uiEnable/1 -> Bus Creator/1  "uiEnable"

== system QiMotorController_ModelReference/Simulation Controls/tiltMotor ==
  note: 1: Current controller
      | 2: Speed controller
      | 3: Position controller
  Bus Creator : BusCreator  Inputs=7
  tiltMotor_OneOverSensorPolepairs : Constant  OutDataTypeStr=single  SampleTime=-1
  tiltMotor_TiltReadheadCompensationEnabled : Constant  Value=0  OutDataTypeStr=int32  SampleTime=-1
  tiltMotor_controlSelector : Constant  Value=3  OutDataTypeStr=uint32  SampleTime=-1
  tiltMotor_currentSetpoint : Constant  Value=0.5  OutDataTypeStr=single  SampleTime=-1
  tiltMotor_positionSetpoint : Step  Time=1.5  Before=pi/30  After=-pi/40  OutDataTypeStr=single
  tiltMotor_speedSetpoint : Constant  Value=200  OutDataTypeStr=single  SampleTime=-1
  tiltMotor_uiEnable : Constant  OutDataTypeStr=uint32  SampleTime=-1
  Out1 : Outport
  wires:
  Bus Creator/1 -> Out1/1  "tiltMotor_simControls"
  tiltMotor_uiEnable/1 -> Bus Creator/1  "uiEnable"
  tiltMotor_controlSelector/1 -> Bus Creator/2  "controlSelector"
  tiltMotor_currentSetpoint/1 -> Bus Creator/3  "currentSetpoint"
  tiltMotor_positionSetpoint/1 -> Bus Creator/5  "positionSetpoint"
  tiltMotor_speedSetpoint/1 -> Bus Creator/4  "speedSetpoint"
  tiltMotor_OneOverSensorPolepairs/1 -> Bus Creator/6  "OneOverSensorPolePairs"
  tiltMotor_TiltReadheadCompensationEnabled/1 -> Bus Creator/7  "TiltReadheadCompensationEnabled"
